simulink model "controlledForwardResponse"  (R2024b)
settings: Solver=VariableStepAuto  StartTime=0.0  StopTime=3  RelTol=1e-3
values from neighbouring files (symbols this model uses):
  K = .65    (= 0.65)    [runControlledForwardResponse.m]    (also in runForwardResponse.m = 0.17)
  kp = 6.5    [runControlledForwardResponse.m]
  sigma = 11    [runControlledForwardResponse.m]    (also in runForwardResponse.m = 10)
libraries: simulink x1
settings Model: Creator=iankeeffe  LastModifiedBy=iankeeffe

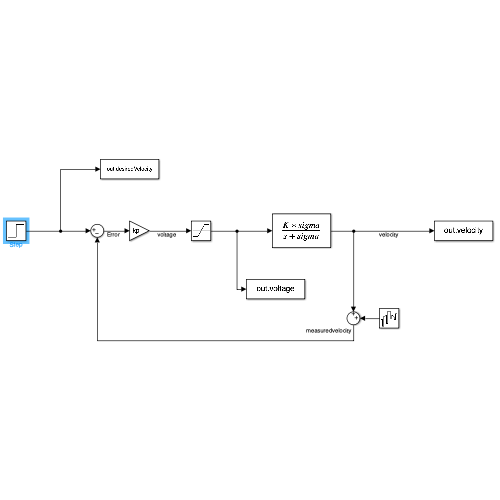
[thumbnail: Simulink's stored preview of the top-level diagram]
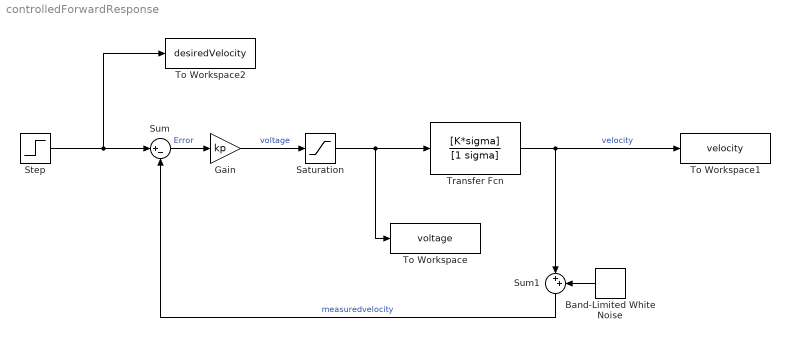
== system controlledForwardResponse ==
  Band-Limited White Noise : simulink/Sources/Band-Limited White Noise  Cov=[0.0001]  Ts=0.01  seed=[23341]
  Gain : Gain  Gain=kp
  Saturation : Saturate  UpperLimit=15  LowerLimit=-15
  Step : Step  SampleTime=0
  Sum : Sum  Inputs=|+-
  Sum1 : Sum  Inputs=|++
  To Workspace : ToWorkspace  VariableName=voltage  SaveFormat=Timeseries  SampleTime=-1
  To Workspace1 : ToWorkspace  VariableName=velocity  SaveFormat=Timeseries  SampleTime=-1
  To Workspace2 : ToWorkspace  VariableName=desiredVelocity  SaveFormat=Timeseries  SampleTime=-1
  Transfer Fcn : TransferFcn  Numerator=[K*sigma]  Denominator=[1 sigma]
  wires:
  Gain/1 -> Saturation/1  "voltage"
  Transfer Fcn/1 -> To Workspace1/1, Sum1/1  "velocity"
  Sum/1 -> Gain/1  "Error"
  Step/1 -> To Workspace2/1, Sum/1
  Saturation/1 -> To Workspace/1, Transfer Fcn/1
  Sum1/1 -> Sum/2  "measuredvelocity"
  Band-Limited White Noise/1 -> Sum1/2
